simulink library "INP_IMU_ManOverAngRat2"  (R2024b)
settings: Solver=VariableStepAuto  StartTime=0.0  StopTime=10.0  RelTol=1e-3
undefined symbols (not defined in the file): INP_IMU_p_AngRatPitchVehLoLim_radps, INP_IMU_p_AngRatPitchVehMan_radps, INP_IMU_p_AngRatPitchVehUpLim_radps, INP_IMU_p_AngRatRollVehLoLim_radps, INP_IMU_p_AngRatRollVehMan_radps, INP_IMU_p_AngRatRollVehUpLim_radps, INP_IMU_p_AngRatYawVehLoLim_radps, INP_IMU_p_AngRatYawVehMan_radps, INP_IMU_p_AngRatYawVehUpLim_radps, INP_IMU_p_SwtAngRatPitchVehMan_na, INP_IMU_p_SwtAngRatRollVehMan_na, INP_IMU_p_SwtAngRatYawVehMan_na
libraries: simulink x3
settings Model: Creator=blatak  LastModifiedBy=jmbsp
settings RTWCC: GPUComputeCapability=3.5

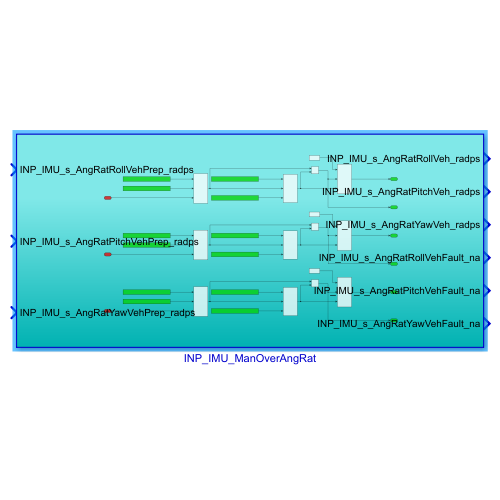
[thumbnail: Simulink's stored preview of the top-level diagram]
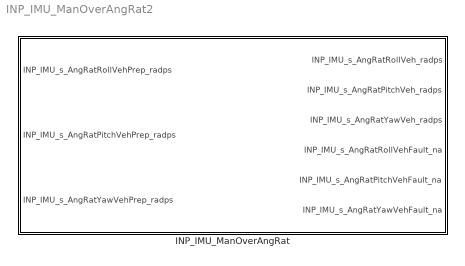
== system INP_IMU_ManOverAngRat2 ==
  INP_IMU_ManOverAngRat : Subsystem  Description=Manual override of measured value (some default value replaces the measured one) and saturation

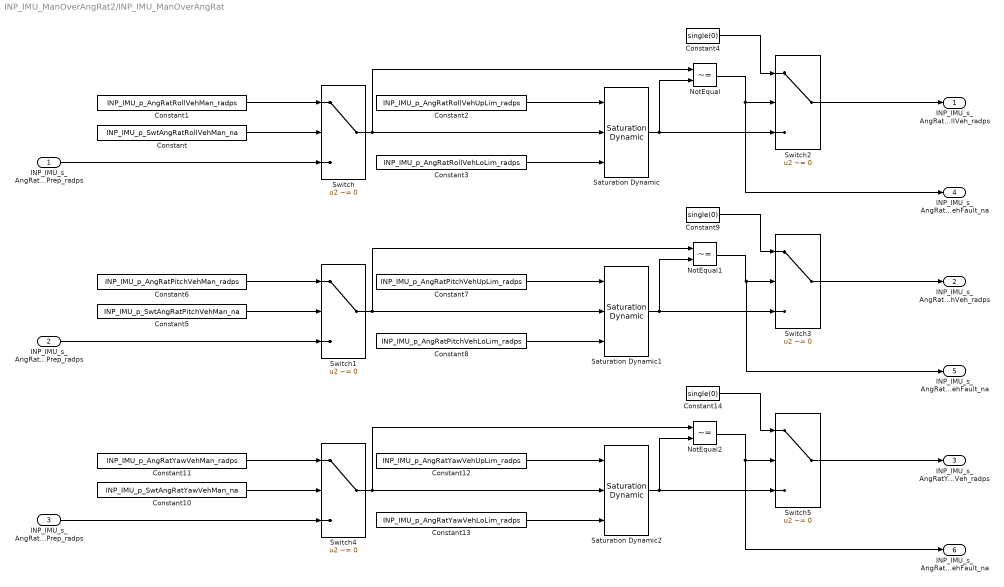
== system INP_IMU_ManOverAngRat2/INP_IMU_ManOverAngRat ==
  INP_IMU_s_AngRatRollVehPrep_radps : Inport  Description=IMU Angular roll velocity - prepared - scale, offset, filtering
  INP_IMU_s_AngRatPitchVehPrep_radps : Inport  Description=IMU Angular pitch velocity - prepared - scale, offset, filtering  Port=2
  INP_IMU_s_AngRatYawVehPrep_radps : Inport  Description=IMU Angular yaw velocity - prepared - scale, offset, filtering  Port=3
  Constant : Constant  Description=|  Value=INP_IMU_p_SwtAngRatRollVehMan_na
      | Switch for manual override of the roll velocity value, if 1 instead the measured 
      | value the INP_IMU_p_AngRatXxxVehMan_radps is used
  Constant1 : Constant  Description=|  Value=INP_IMU_p_AngRatRollVehMan_radps
      | Value for roll velocity, which is used if the INP_IMU_p_SwtAngRatXxxVehMan_na
      | is set to 1 instead of the measured value
  Constant10 : Constant  Description=|  Value=INP_IMU_p_SwtAngRatYawVehMan_na
      | Switch for manual override of the yaw velocity value, if 1 instead the measured 
      | value the INP_IMU_p_AngRatXxxVehMan_radps is used
  Constant11 : Constant  Description=|  Value=INP_IMU_p_AngRatYawVehMan_radps
      | Value for yaw velocity, which is used if the INP_IMU_p_SwtAngRatXxxVehMan_na
      | is set to 1 instead of the measured value
  Constant12 : Constant  Description=Upper saturation limit for yaw velocity  Value=INP_IMU_p_AngRatYawVehUpLim_radps
  Constant13 : Constant  Description=Lower saturation limit for yaw velocity  Value=INP_IMU_p_AngRatYawVehLoLim_radps
  Constant14 : Constant  Value=single(0)
  Constant2 : Constant  Description=Upper saturation limit for roll velocity  Value=INP_IMU_p_AngRatRollVehUpLim_radps
  Constant3 : Constant  Description=Lower saturation limit for roll velocity  Value=INP_IMU_p_AngRatRollVehLoLim_radps
  Constant4 : Constant  Value=single(0)
  Constant5 : Constant  Description=|  Value=INP_IMU_p_SwtAngRatPitchVehMan_na
      | Switch for manual override of the pitch velocity value, if 1 instead the measured 
      | value the INP_IMU_p_AngRatXxxVehMan_radps is used
  Constant6 : Constant  Description=|  Value=INP_IMU_p_AngRatPitchVehMan_radps
      | Value for pitch velocity, which is used if the INP_IMU_p_SwtAngRatXxxVehMan_na
      | is set to 1 instead of the measured value
  Constant7 : Constant  Description=Upper saturation limit for pitch velocity  Value=INP_IMU_p_AngRatPitchVehUpLim_radps
  Constant8 : Constant  Description=Lower saturation limit for pitch velocity  Value=INP_IMU_p_AngRatPitchVehLoLim_radps
  Constant9 : Constant  Value=single(0)
  NotEqual : RelationalOperator  Operator=~=  OutDataTypeStr=boolean  RndMeth=Simplest  InputSameDT=off
  NotEqual1 : RelationalOperator  Operator=~=  OutDataTypeStr=boolean  RndMeth=Simplest  InputSameDT=off
  NotEqual2 : RelationalOperator  Operator=~=  OutDataTypeStr=boolean  RndMeth=Simplest  InputSameDT=off
  Saturation Dynamic : simulink/Discontinuities/Saturation Dynamic  OutMin=[]  OutMax=[]  OutDataTypeStr=Inherit: Same as second input  OutDataType=fixdt(1, 16)  OutScaling=2^-10  DoSatur=off
  Saturation Dynamic1 : simulink/Discontinuities/Saturation Dynamic  OutMin=[]  OutMax=[]  OutDataTypeStr=Inherit: Same as second input  OutDataType=fixdt(1, 16)  OutScaling=2^-10  DoSatur=off
  Saturation Dynamic2 : simulink/Discontinuities/Saturation Dynamic  OutMin=[]  OutMax=[]  OutDataTypeStr=Inherit: Same as second input  OutDataType=fixdt(1, 16)  OutScaling=2^-10  DoSatur=off
  Switch{,1..5} (6 alike) : Switch  Criteria=u2 ~= 0  SaturateOnIntegerOverflow=off  InputSameDT=off
  INP_IMU_s_AngRatRollVeh_radps : Outport  Description=INP IMU Vehicle angular roll velocity - manual override, saturation
  INP_IMU_s_AngRatPitchVeh_radps : Outport  Description=INP IMU Vehicle angular pitch velocity - manual override, saturation  Port=2
  INP_IMU_s_AngRatYawVeh_radps : Outport  Description=INP IMU Vehicle angular yaw velocity - manual override, saturation  Port=3
  INP_IMU_s_AngRatRollVehFault_na : Outport  Port=4
  INP_IMU_s_AngRatPitchVehFault_na : Outport  Port=5
  INP_IMU_s_AngRatYawVehFault_na : Outport  Port=6
  wires:
  Constant8/1 -> Saturation Dynamic1/3
  INP_IMU_s_AngRatYawVehPrep_radps/1 -> Switch4/3
  NotEqual2/1 -> INP_IMU_s_AngRatYawVehFault_na/1, Switch5/2
  Constant11/1 -> Switch4/1
  NotEqual/1 -> INP_IMU_s_AngRatRollVehFault_na/1, Switch2/2
  Switch2/1 -> INP_IMU_s_AngRatRollVeh_radps/1
  Constant/1 -> Switch/2
  Saturation Dynamic2/1 -> NotEqual2/2, Switch5/3
  Switch1/1 -> Saturation Dynamic1/2, NotEqual1/1
  Constant12/1 -> Saturation Dynamic2/1
  Switch5/1 -> INP_IMU_s_AngRatYawVeh_radps/1
  Constant13/1 -> Saturation Dynamic2/3
  Constant4/1 -> Switch2/1
  Constant10/1 -> Switch4/2
  Constant1/1 -> Switch/1
  NotEqual1/1 -> INP_IMU_s_AngRatPitchVehFault_na/1, Switch3/2
  Saturation Dynamic1/1 -> NotEqual1/2, Switch3/3
  Constant5/1 -> Switch1/2
  Constant14/1 -> Switch5/1
  INP_IMU_s_AngRatPitchVehPrep_radps/1 -> Switch1/3
  Switch4/1 -> Saturation Dynamic2/2, NotEqual2/1
  Constant3/1 -> Saturation Dynamic/3
  Switch3/1 -> INP_IMU_s_AngRatPitchVeh_radps/1
  Switch/1 -> Saturation Dynamic/2, NotEqual/1
  Saturation Dynamic/1 -> NotEqual/2, Switch2/3
  Constant6/1 -> Switch1/1
  Constant2/1 -> Saturation Dynamic/1
  Constant7/1 -> Saturation Dynamic1/1
  INP_IMU_s_AngRatRollVehPrep_radps/1 -> Switch/3
  Constant9/1 -> Switch3/1
